simulink model "Boomerang_dihedral_simulink"  (R2023a)
settings: Solver=ode4  StartTime=0.0  StopTime=t  FixedStep=dt  MaxStep=maxstep  MinStep=minstep
values from neighbouring files (symbols this model uses):
  betaj = deg2rad(betaj)    [SmartBoomerang_Sim.m]
  c = 5e-2    (= 0.05)    [SmartBoomerang_Sim.m]
  CDdata = [x_CD, y_CD]    [SmartBoomerang_Sim.m]
  CLdata = [x_CL, y_CL]    [SmartBoomerang_Sim.m]
  CMdata = [x_CM, y_CM]    [SmartBoomerang_Sim.m]
  Eul0 = [0; 0; 0]    [SmartBoomerang_Sim.m]
  g = 9.81    [SmartBoomerang_Sim.m]
  gamma = deg2rad(gamma)    [SmartBoomerang_Sim.m]
  invTI0 = transpose(TI0)    [SmartBoomerang_Sim.m]
  J = J + (Ji(:,:,i))    [SmartBoomerang_Sim.m]
  Jj = [ ... (first row only)    [SmartBoomerang_Sim.m]
  Kd = 1    [SmartBoomerang_Sim.m]
  Ki = 0    [SmartBoomerang_Sim.m]
  Kp = 0.5    [SmartBoomerang_Sim.m]
  l_integrate = linspace(0,l_blade,n)    [SmartBoomerang_Sim.m]
  LAMBDAj = deg2rad(LAMBDAj)    [SmartBoomerang_Sim.m]
  m = 200e-3    (= 0.2)    [SmartBoomerang_Sim.m]
  max_dd = deg2rad(max_dd)    [SmartBoomerang_Sim.m]
  min_dd = deg2rad(min_dd)    [SmartBoomerang_Sim.m]
  n = n + 1    (= 51)    [SmartBoomerang_Sim.m]
  nw = 4    [SmartBoomerang_Sim.m]
  omega0 = [0; 0; 10*pi*2]    [SmartBoomerang_Sim.m]
  R_pos0 = [0; 0; 1.5]    [SmartBoomerang_Sim.m]
  rho = 1.22    [SmartBoomerang_Sim.m]
  S = pi*R^2    (= 0.196349540849)    [SmartBoomerang_Sim.m]
  servo_rpm = deg2rad(servo_rpm)    [SmartBoomerang_Sim.m]
  thetaj = 0    [SmartBoomerang_Sim.m]
  TI0 = RI01*RI02*RI03    [SmartBoomerang_Sim.m]
  u0 = TI0*U0    [SmartBoomerang_Sim.m]
  v_wind = [0; 1.5; 0]    [SmartBoomerang_Sim.m]
  x_ac = zeros(3,nw)    [SmartBoomerang_Sim.m]
  X_des = [x_des, y_des]    [SmartBoomerang_Sim.m]
settings Model: Creator=dsantis  LastModifiedBy=dsantis

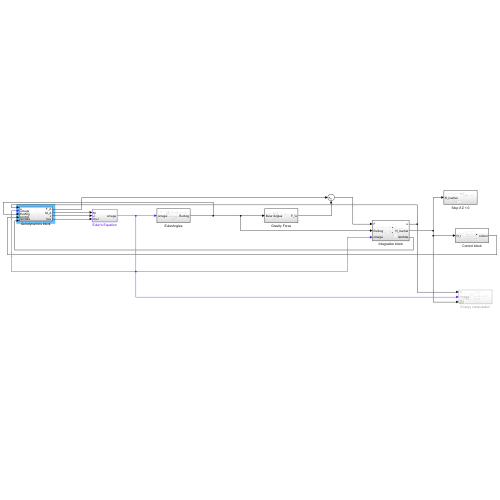
[thumbnail: Simulink's stored preview of the top-level diagram]
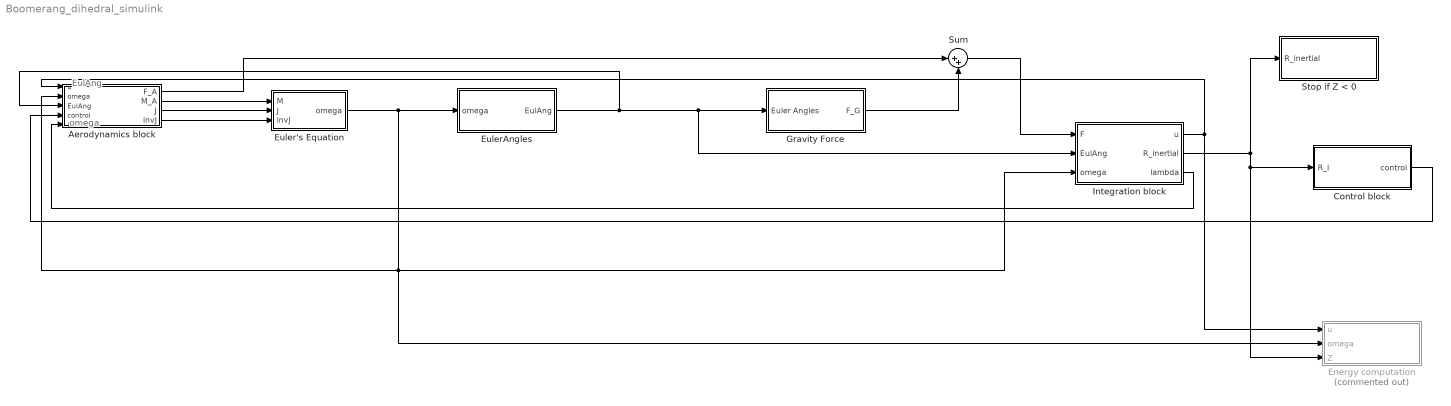
== system Boomerang_dihedral_simulink ==
  note: omega
  note: EulAng
  Aerodynamics block : Subsystem
  Control block : Subsystem
  Energy computation : Subsystem  Commented=on
  Euler's Equation : Subsystem
  EulerAngles : Subsystem
  Gravity Force : Subsystem
  Integration block : Subsystem
  Stop if Z < 0 : Subsystem
  Sum : Sum  Inputs=|++
  wires:
  Sum/1 -> Integration block/1(F)
  Control block/1(control) -> Aerodynamics block/4(control)
  Gravity Force/1(F_G) -> Sum/2
  Aerodynamics block/4(invJ) -> Euler's Equation/3(invJ)
  Aerodynamics block/3(J) -> Euler's Equation/2(J)
  Aerodynamics block/2(M_A) -> Euler's Equation/1(M)
  Integration block/2(R_inertial) -> Control block/1(R_I), Energy computation/3(Z), Stop if Z < 0/1(R_inertial)
  Euler's Equation/1(omega) -> Energy computation/2(omega), Aerodynamics block/2(omega), Integration block/3(omega), EulerAngles/1(omega)
  Aerodynamics block/1(F_A) -> Sum/1
  Integration block/1(u) -> Energy computation/1(u), Aerodynamics block/1(u)
  EulerAngles/1(EulAng) -> Integration block/2(EulAng), Gravity Force/1(Euler Angles), Aerodynamics block/3(EulAng)
  Integration block/3(lambda) -> Aerodynamics block/5(lambda)

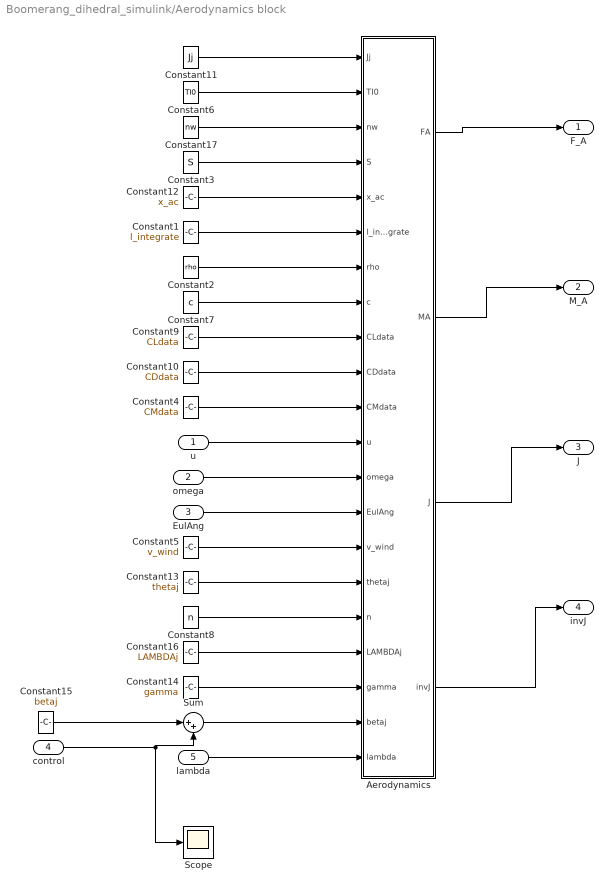
== system Boomerang_dihedral_simulink/Aerodynamics block ==
  u : Inport
  omega : Inport  Port=2
  EulAng : Inport  Port=3
  control : Inport  Port=4
  lambda : Inport  Port=5
  Aerodynamics : MATLAB Function  TreatAsAtomicUnit=on
  Constant1 : Constant  Value=l_integrate
  Constant10 : Constant  Value=CDdata
  Constant11 : Constant  Value=Jj
  Constant12 : Constant  Value=x_ac
  Constant13 : Constant  Value=thetaj
  Constant14 : Constant  Value=gamma
  Constant15 : Constant  Value=betaj
  Constant16 : Constant  Value=LAMBDAj
  Constant17 : Constant  Value=nw
  Constant2 : Constant  Value=rho
  Constant3 : Constant  Value=S
  Constant4 : Constant  Value=CMdata
  Constant5 : Constant  Value=v_wind
  Constant6 : Constant  Value=TI0
  Constant7 : Constant  Value=c
  Constant8 : Constant  Value=n
  Constant9 : Constant  Value=CLdata
  Scope : Scope
  Sum : Sum  Inputs=|++
  F_A : Outport
  M_A : Outport  Port=2
  J : Outport  Port=3
  invJ : Outport  Port=4
  wires:
  u/1 -> Aerodynamics/12(u)
  Constant2/1 -> Aerodynamics/7(rho)
  Constant9/1 -> Aerodynamics/9(CLdata)
  Constant10/1 -> Aerodynamics/10(CDdata)
  Constant1/1 -> Aerodynamics/6(l_integrate)
  Constant7/1 -> Aerodynamics/8(c)
  omega/1 -> Aerodynamics/13(omega)
  Constant17/1 -> Aerodynamics/3(nw)
  Constant3/1 -> Aerodynamics/4(S)
  Aerodynamics/1(FA) -> F_A/1
  Constant4/1 -> Aerodynamics/11(CMdata)
  Aerodynamics/2(MA) -> M_A/1
  EulAng/1 -> Aerodynamics/14(EulAng)
  Constant5/1 -> Aerodynamics/15(v_wind)
  Constant6/1 -> Aerodynamics/2(TI0)
  Constant8/1 -> Aerodynamics/17(n)
  Aerodynamics/3(J) -> J/1
  Aerodynamics/4(invJ) -> invJ/1
  Constant11/1 -> Aerodynamics/1(Jj)
  Constant13/1 -> Aerodynamics/16(thetaj)
  control/1 -> Scope/1, Sum/2
  Constant12/1 -> Aerodynamics/5(x_ac)
  Sum/1 -> Aerodynamics/20(betaj)
  Constant14/1 -> Aerodynamics/19(gamma)
  Constant15/1 -> Sum/1
  Constant16/1 -> Aerodynamics/18(LAMBDAj)
  lambda/1 -> Aerodynamics/21(lambda)

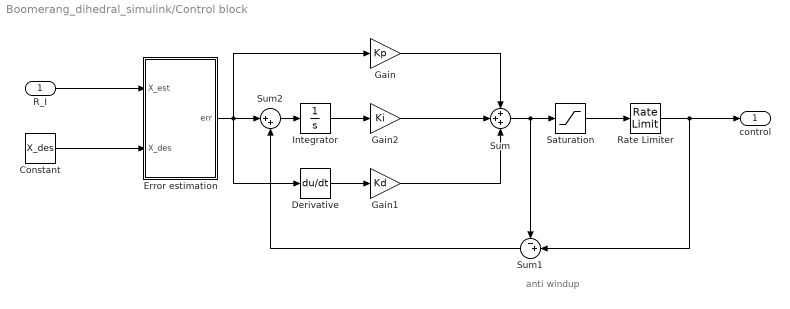
== system Boomerang_dihedral_simulink/Control block ==
  note: anti windup
  R_I : Inport
  Constant : Constant  Value=X_des
  Derivative : Derivative
  Error estimation : MATLAB Function  TreatAsAtomicUnit=on
  Gain : Gain  Gain=Kp
  Gain1 : Gain  Gain=Kd
  Gain2 : Gain  Gain=Ki
  Integrator : Integrator  LimitOutput=on  UpperSaturationLimit=pi/Ki  LowerSaturationLimit=-pi/Ki
  Rate Limiter : RateLimiter  RisingSlewLimit=servo_rpm  FallingSlewLimit=-servo_rpm  SampleTimeMode=inherited
  Saturation : Saturate  UpperLimit=max_dd  LowerLimit=min_dd
  Sum : Sum  Inputs=+++
  Sum1 : Sum  Inputs=-+|
  Sum2 : Sum  Inputs=|++
  control : Outport
  wires:
  R_I/1 -> Error estimation/1(X_est)
  Constant/1 -> Error estimation/2(X_des)
  Error estimation/1(err) -> Sum2/1, Derivative/1, Gain/1
  Gain/1 -> Sum/1
  Derivative/1 -> Gain1/1
  Gain1/1 -> Sum/3
  Saturation/1 -> Rate Limiter/1
  Rate Limiter/1 -> Sum1/2, control/1
  Integrator/1 -> Gain2/1
  Gain2/1 -> Sum/2
  Sum2/1 -> Integrator/1
  Sum1/1 -> Sum2/2
  Sum/1 -> Saturation/1, Sum1/1

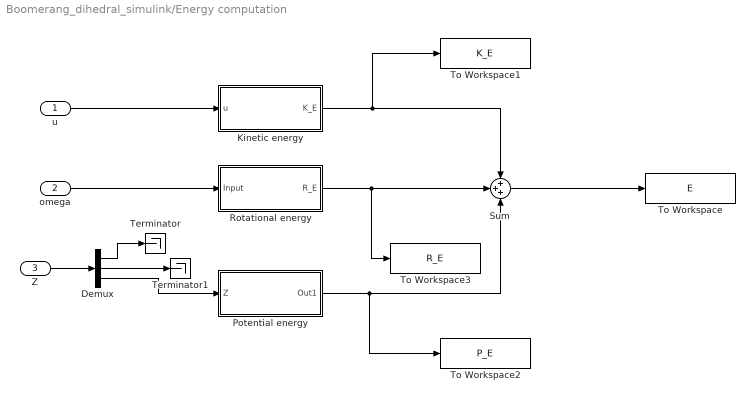
== system Boomerang_dihedral_simulink/Energy computation ==
  u : Inport
  omega : Inport  Port=2
  Z : Inport  Port=3
  Demux : Demux  Outputs=3
  Kinetic energy : Subsystem
  Potential energy : Subsystem
  Rotational energy : Subsystem
  Sum : Sum  Inputs=+++
  Terminator : Terminator
  Terminator1 : Terminator
  To Workspace : ToWorkspace  VariableName=E  SaveFormat=Timeseries  SampleTime=-1
  To Workspace1 : ToWorkspace  VariableName=K_E  SaveFormat=Timeseries  SampleTime=-1
  To Workspace2 : ToWorkspace  VariableName=P_E  SaveFormat=Timeseries  SampleTime=-1
  To Workspace3 : ToWorkspace  VariableName=R_E  SaveFormat=Timeseries  SampleTime=-1
  wires:
  u/1 -> Kinetic energy/1(u)
  omega/1 -> Rotational energy/1(Input)
  Z/1 -> Demux/1
  Demux/3 -> Potential energy/1(Z)
  Demux/1 -> Terminator/1
  Demux/2 -> Terminator1/1
  Kinetic energy/1(K_E) -> To Workspace1/1, Sum/1
  Rotational energy/1(R_E) -> To Workspace3/1, Sum/2
  Potential energy/1(Out1) -> To Workspace2/1, Sum/3
  Sum/1 -> To Workspace/1

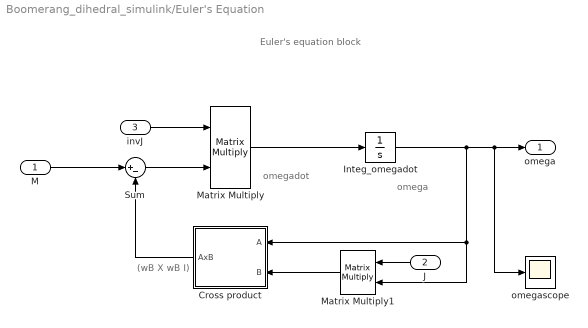
== system Boomerang_dihedral_simulink/Euler's Equation ==
  note: Euler's equation block
  note: (wB X wB I)
  note: omega
  note: omegadot
  M : Inport
  J : Inport  Port=2
  invJ : Inport  Port=3
  Cross product : Subsystem
  Integ_omegadot : Integrator  InitialCondition=omega0
  Matrix Multiply : Product  Multiplication=Matrix(*)
  Matrix Multiply1 : Product  Multiplication=Matrix(*)
  Sum : Sum  Inputs=|+-
  omegascope : Scope
  omega : Outport  VectorParamsAs1DForOutWhenUnconnected=off
  wires:
  Integ_omegadot/1 -> Cross product/1(A), Matrix Multiply1/2, omegascope/1, omega/1
  Matrix Multiply1/1 -> Cross product/2(B)
  M/1 -> Sum/1
  Sum/1 -> Matrix Multiply/2
  Matrix Multiply/1 -> Integ_omegadot/1
  Cross product/1(AxB) -> Sum/2
  invJ/1 -> Matrix Multiply/1
  J/1 -> Matrix Multiply1/1

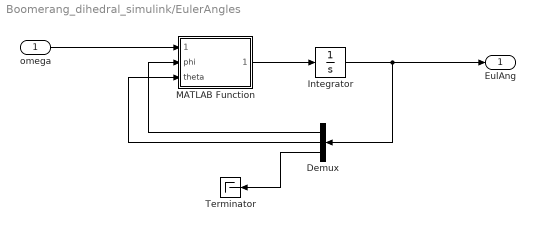
== system Boomerang_dihedral_simulink/EulerAngles ==
  omega : Inport
  Demux : Demux  Outputs=3
  Integrator : Integrator  InitialCondition=Eul0
  MATLAB Function : MATLAB Function  TreatAsAtomicUnit=on
  Terminator : Terminator
  EulAng : Outport
  wires:
  omega/1 -> MATLAB Function/1(omega)
  MATLAB Function/1(EulRate) -> Integrator/1
  Integrator/1 -> Demux/1, EulAng/1
  Demux/1 -> MATLAB Function/2(phi)
  Demux/2 -> MATLAB Function/3(theta)
  Demux/3 -> Terminator/1

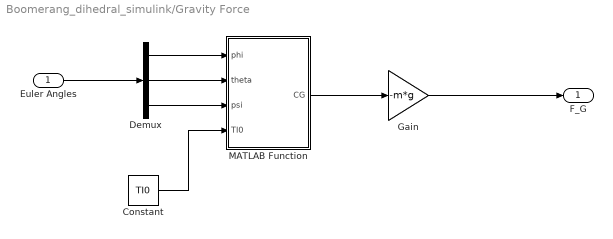
== system Boomerang_dihedral_simulink/Gravity Force ==
  Euler Angles : Inport
  Constant : Constant  Value=TI0
  Demux : Demux  Outputs=3
  Gain : Gain  Gain=-m*g
  MATLAB Function : MATLAB Function  TreatAsAtomicUnit=on
  F_G : Outport
  wires:
  Gain/1 -> F_G/1
  Demux/3 -> MATLAB Function/3(psi)
  Demux/2 -> MATLAB Function/2(theta)
  Demux/1 -> MATLAB Function/1(phi)
  MATLAB Function/1(CG) -> Gain/1
  Euler Angles/1 -> Demux/1
  Constant/1 -> MATLAB Function/4(TI0)

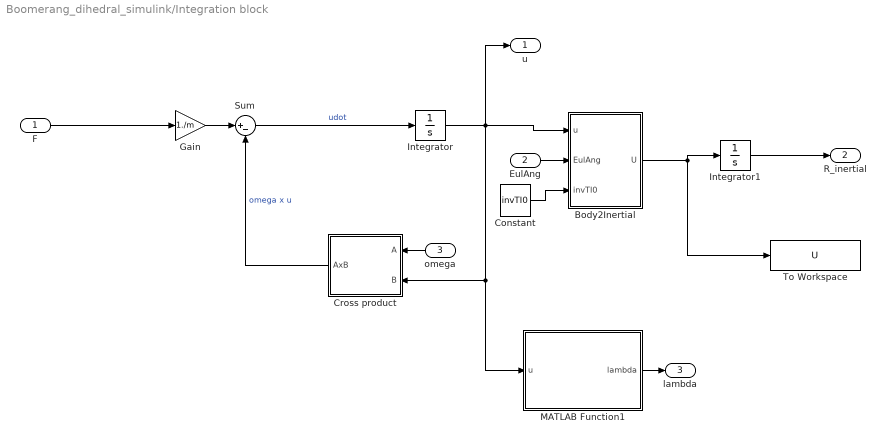
== system Boomerang_dihedral_simulink/Integration block ==
  F : Inport
  EulAng : Inport  Port=2
  omega : Inport  Port=3
  Body2Inertial : MATLAB Function  TreatAsAtomicUnit=on
  Constant : Constant  Value=invTI0
  Cross product : Subsystem
  Gain : Gain  Gain=1./m
  Integrator : Integrator  InitialCondition=u0
  Integrator1 : Integrator  InitialCondition=R_pos0
  MATLAB Function1 : MATLAB Function  TreatAsAtomicUnit=on
  Sum : Sum  Inputs=|+-
  To Workspace : ToWorkspace  VariableName=U  SampleTime=-1
  u : Outport
  R_inertial : Outport  Port=2
  lambda : Outport  Port=3
  wires:
  Cross product/1(AxB) -> Sum/2  "omega x u"
  Integrator/1 -> MATLAB Function1/1(u), Cross product/2(B), Body2Inertial/1(u), u/1
  Integrator1/1 -> R_inertial/1
  Gain/1 -> Sum/1
  EulAng/1 -> Body2Inertial/2(EulAng)
  Constant/1 -> Body2Inertial/3(invTI0)
  F/1 -> Gain/1
  Body2Inertial/1(U) -> Integrator1/1, To Workspace/1
  omega/1 -> Cross product/1(A)
  Sum/1 -> Integrator/1  "udot"
  MATLAB Function1/1(lambda) -> lambda/1

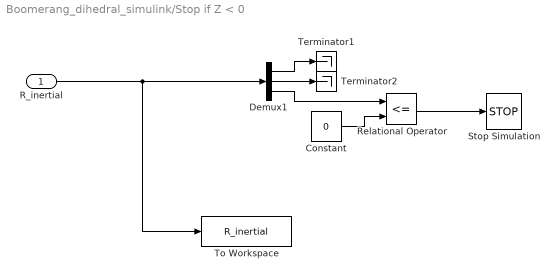
== system Boomerang_dihedral_simulink/Stop if Z < 0 ==
  R_inertial : Inport
  Constant : Constant  Value=0
  Demux1 : Demux  Outputs=3
  Relational Operator : RelationalOperator  Operator=<=  OutDataTypeStr=boolean  RndMeth=Simplest  InputSameDT=off
  Stop Simulation : Stop
  Terminator1 : Terminator
  Terminator2 : Terminator
  To Workspace : ToWorkspace  VariableName=R_inertial  SampleTime=-1
  wires:
  R_inertial/1 -> To Workspace/1, Demux1/1
  Demux1/1 -> Terminator1/1
  Demux1/3 -> Relational Operator/1
  Demux1/2 -> Terminator2/1
  Constant/1 -> Relational Operator/2
  Relational Operator/1 -> Stop Simulation/1

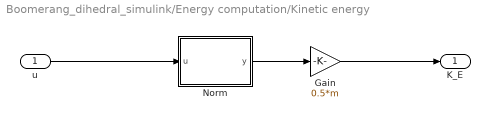
== system Boomerang_dihedral_simulink/Energy computation/Kinetic energy ==
  u : Inport
  Gain : Gain  Gain=0.5*m
  Norm : MATLAB Function  TreatAsAtomicUnit=on
  K_E : Outport
  wires:
  u/1 -> Norm/1(u)
  Norm/1(y) -> Gain/1
  Gain/1 -> K_E/1

== system Boomerang_dihedral_simulink/Energy computation/Potential energy ==
  Z : Inport
  Gain : Gain  Gain=m*g
  Out1 : Outport
  wires:
  Z/1 -> Gain/1
  Gain/1 -> Out1/1

== system Boomerang_dihedral_simulink/Energy computation/Rotational energy ==
  Input : Inport
  Dot Product : DotProduct  OutDataTypeStr=Inherit: Inherit via internal rule
  Gain : Gain  Gain=0.5*J  Multiplication=Matrix(u*K)
  R_E : Outport
  wires:
  Input/1 -> Dot Product/2, Gain/1
  Gain/1 -> Dot Product/1
  Dot Product/1 -> R_E/1

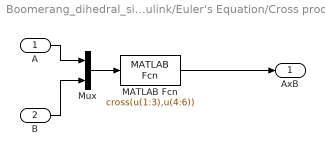
== system Boomerang_dihedral_simulink/Euler's Equation/Cross product ==
  A : Inport
  B : Inport  Port=2
  MATLAB Fcn : MATLABFcn  MATLABFcn=cross(u(1:3),u(4:6))
  Mux : Mux  Inputs=2
  AxB : Outport  VectorParamsAs1DForOutWhenUnconnected=off
  wires:
  A/1 -> Mux/1
  B/1 -> Mux/2
  Mux/1 -> MATLAB Fcn/1
  MATLAB Fcn/1 -> AxB/1

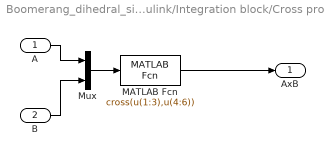
== system Boomerang_dihedral_simulink/Integration block/Cross product ==
  A : Inport
  B : Inport  Port=2
  MATLAB Fcn : MATLABFcn  MATLABFcn=cross(u(1:3),u(4:6))
  Mux : Mux  Inputs=2
  AxB : Outport  VectorParamsAs1DForOutWhenUnconnected=off
  wires:
  A/1 -> Mux/1
  B/1 -> Mux/2
  Mux/1 -> MATLAB Fcn/1
  MATLAB Fcn/1 -> AxB/1

== matlab function Boomerang_dihedral_simulink/Control block/Error estimation ==
  settings: updateMethod=DISCRETE
  data: X_est input; err output; X_des input
function err = fcn(X_est,X_des)

persistent i_old % Having i as a persistent variable allows to look for the closest distance between the boomerang and the reference path;
% This way, the final target will always be the final point of the
% returning path (the thrower)
if isempty(i_old)
    i_old = 1;
end

% Find which desired trajectory point is nearest to the boomerang and
% compute the error. 
X_des = X_des(i_old:end,1:2);

[err_vec, i] = min(vecnorm([X_est(1), X_est(2)] - X_des,2,2));

% Figure out if you are to the left or to the right of the desired
% trajectory in order to determine the sign of the error and follow with
% the proper control maneuver
err_sign = sign(norm([X_est(1), X_est(2)]) - norm([X_des(i,1), X_des(i,2)]));

err = err_sign*err_vec;
% if err_sign == -1
%     if abs(err) < 1
%         err = 0;
%     end
% end

i_old = i_old + i - 1;

end

== matlab function Boomerang_dihedral_simulink/Energy computation/Kinetic energy/Norm ==
  data: u input; y output
function y = fcn(u)

y = norm(u)^2;

== matlab function Boomerang_dihedral_simulink/Integration block/MATLAB Function1 ==
  data: u input; lambda output
function lambda = fcn(u)

ux = u(1);
uy = u(2);

lambda = -atan2(uy,ux);

== matlab function Boomerang_dihedral_simulink/Aerodynamics block/Aerodynamics ==
  settings: updateMethod=DISCRETE
  data: Jj input; TI0 input; nw input; S input; x_ac input; l_integrate input; rho input; c input; CLdata input; CDdata input; CMdata input; u input; omega input; EulAng input; v_wind input; FA output; thetaj input; MA output; n input; LAMBDAj input; J output; invJ output; gamma input; betaj input; lambda input
function [FA, MA, J, invJ] = fcn(Jj, TI0, nw, S, x_ac, l_integrate, rho, c, CLdata, CDdata, CMdata,u, omega, EulAng, v_wind, thetaj, n, LAMBDAj, gamma, betaj, lambda)
phi = EulAng(1);
theta = EulAng(2);
psi = EulAng(3);

R01 = [1, 0, 0; 0, cos(phi), sin(phi); 0, -sin(phi), cos(phi)];
R02 = [cos(theta), 0, -sin(theta); 0, 1, 0; sin(theta), 0, cos(theta)];
R03 = [cos(psi), sin(psi), 0; -sin(psi), cos(psi), 0; 0, 0, 1];
T0 = R01*R02*R03;

Tj = zeros(3,3, nw);
invTj = zeros(3,3,nw);

for i = 0:(nw-1)
Rj1 = [1, 0, 0; 0, cos(betaj), sin(betaj); 0, -sin(betaj), cos(betaj)];
    Rj2 = [cos(thetaj), 0, -sin(thetaj);0, 1, 0; sin(thetaj), 0, cos(thetaj)];
    Rj3 = [cos(LAMBDAj-pi/2 + gamma*i), sin(LAMBDAj-pi/2 + gamma*i), 0; ...
        -sin(LAMBDAj-pi/2 + gamma*i), cos(LAMBDAj-pi/2+ gamma*i), 0;0, 0, 1];
    Tj(:,:,i+1) = Rj2*Rj1*Rj3;
    invTj(:,:,i+1) = transpose(Tj(:,:,i+1));
end
Ji = zeros(3,3,nw);
J = zeros(3);
for i = 1:nw
    Ji(:,:,i) = invTj(:,:,i)*Jj*Tj(:,:,i);
    J = J + (Ji(:,:,i));
end
% J = diag(diag(J));

invJ = inv(J);
r = l_integrate./l_integrate(end);

persistent flag v_bar
if isempty(flag)
    flag = false;
    v_bar = 0;
end

% Piecewise linear fit for CL
C_L = @(alpha) interp1(CLdata(:,1), CLdata(:,2), alpha, 'linear', 'extrap');

% Piecewise linear fit for CD
C_D = @(alpha) interp1(CDdata(:,1), CDdata(:,2), alpha, 'linear', 'extrap');

 % Piecewise linear fit for CM
C_M = @(alpha) interp1(CMdata(:,1), CMdata(:,2), alpha, 'linear', 'extrap');

FA = [0; 0; 0];
MA = [0;0;0];

for i = 1:nw
    % Computing induced velocity considering linear variation along the
    % longitudinal direction
    kx = 1.5;
    v_ind = [zeros(size(l_integrate)), zeros(size(l_integrate)), v_bar*(1+kx*cos(lambda + gamma*(i-1))*r)]';

    rA = x_ac(:,i).*ones(3,n) + invTj(:,:,i)*[zeros(1,n); l_integrate'; zeros(1,n)];
    
    w = Tj(:,:,i)*( (-u -cross(omega.*ones(3,n), rA)) + v_ind + T0*TI0*v_wind);
    alpha = (atan2(w(3,:),w(1,:))) + thetaj;
    
    % Computing the tip-loss factor F
    f = abs(nw/2.*(1-r')./(r'.*alpha));
    F =2/pi*acos(exp(-f));

    w2 = w(1,:).^2 + w(3,:).^2;
    
    l = (0.5*rho*c).*w2.*C_L(alpha);
    d = (0.5*rho*c).*w2.*C_D(alpha);
    m_eta = (0.5*rho*c^2).*w2.*C_M(alpha);

    int_funx = F.*(-l.*sin(alpha) + d.*cos(alpha));
    int_funz = (l.*cos(alpha) + d.*sin(alpha));
    
    % int_funMx = (l.*cos(alpha) + d.*sin(alpha)).*l_integrate';
    funM = cross([zeros(1,n); l_integrate'; zeros(1,n)], [int_funx; zeros(1,n); int_funz]);
    int_funMx = funM(1,:);
    int_funMy = m_eta; 
    int_funMz = funM(3,:);
 
    FxjA = trapz(l_integrate,int_funx);
    FzjA = trapz(l_integrate,int_funz);

    MxjA = trapz(l_integrate,int_funMx);
    MyjA = trapz(l_integrate,int_funMy);
    MzjA = trapz(l_integrate,int_funMz);

    FjA = [FxjA; 0; FzjA];
    FA = FA + invTj(:,:,i)*FjA;

    MjA = [MxjA'; MyjA; MzjA];
    MA = MA + invTj(:,:,i)*MjA + cross(x_ac(:,i), invTj(:,:,i)*FjA);

    % WD = WD + 1/2*rho*c*l_integrate(end)*(transpose(invTj(:,:,i)*FjA)*u);
    % WW = WW + 1/2*rho*c*l_integrate(end)*(transpose(invTj(:,:,i)*FjA)*T0*TI0*v_wind);
end
% WD = 1/2*rho*c*l_integrate(end)*FA'*(u + cross(omega,u));
% WW = 1/2*rho*c*l_integrate(end)*FA'*T0*TI0*v_wind;

f = @(v_ind) v_ind - FA(3)/(2*rho*S*sqrt(norm([u(1) u(2)])^2 + (u(3)-v_ind)^2));
v_bar = fzero(f,0);

end

== matlab function Boomerang_dihedral_simulink/Gravity Force/MATLAB Function ==
  data: phi input; theta input; psi input; CG output; TI0 input
function CG = fcn(phi, theta, psi, TI0)
R01 = [
    1, 0, 0;
    0, cos(phi), sin(phi);
    0, -sin(phi), cos(phi)
    ];
R02 = [
    cos(theta), 0, -sin(theta);
    0, 1, 0;
    sin(theta), 0, cos(theta)
];
R03 = [
    cos(psi), sin(psi), 0;
    -sin(psi), cos(psi), 0;
    0, 0, 1
];
T0 = R01*R02*R03;

CG = T0*TI0*[0; 0; 1];

== matlab function Boomerang_dihedral_simulink/Integration block/Body2Inertial ==
  data: u input; U output; EulAng input; invTI0 input
function U = fcn(u, EulAng, invTI0)
phi = EulAng(1);
theta = EulAng(2);
psi = EulAng(3);

R01 = [
    1, 0, 0;
    0, cos(phi), sin(phi);
    0, -sin(phi), cos(phi)
    ];
R02 = [
    cos(theta), 0, -sin(theta);
    0, 1, 0;
    sin(theta), 0, cos(theta)
];
R03 = [
    cos(psi), sin(psi), 0;
    -sin(psi), cos(psi), 0;
    0, 0, 1
];
T0 = R01*R02*R03;
invT0 = transpose(T0);
U = invTI0*invT0*u;

== matlab function Boomerang_dihedral_simulink/EulerAngles/MATLAB Function ==
  data: omega input; EulRate output; phi input; theta input
function EulRate = fcn(omega, phi, theta)

phidot = omega(1) + omega(2)*sin(phi)*tan(theta) + omega(3)*cos(phi)*tan(theta);
thetadot = omega(2)*cos(phi) - omega(3)*sin(phi);
psidot = omega(2)*sin(phi)/cos(theta) + omega(3)*cos(phi)/cos(theta);

EulRate = [phidot; thetadot; psidot];
